simulink model "E3"  (R2020a)
settings: Solver=VariableStepAuto  StartTime=0.0  StopTime=200  RelTol=1e-3
undefined symbols (not defined in the file): c_s, kd, ki, kp
libraries: fl_lib x11, simulink x5, nesl_utility x5
settings Model: Creator=juan  LastModifiedBy=juan

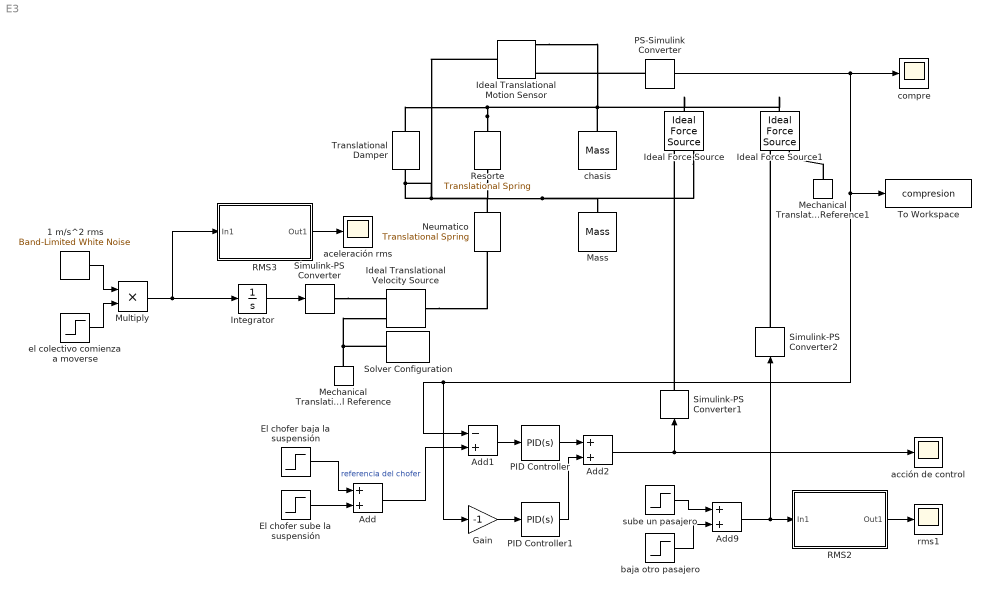
== system E3 ==
  1 m/s^2 rms : simulink/Sources/Band-Limited White Noise  Cov=(1^2)/(1/0.1)  Ts=0.1  seed=[98657]
  Add : Sum
  Add1 : Sum  Inputs=-+
  Add2 : Sum
  Add9 : Sum
  El chofer baja la suspensión : Step  Time=10  After=-0.10  SampleTime=0
  El chofer sube la suspensión : Step  Time=30  After=.10  SampleTime=0
  Gain : Gain  Gain=-1
  Ideal Force Source : fl_lib/Mechanical/Mechanical Sources/Ideal Force Source
  Ideal Force Source1 : fl_lib/Mechanical/Mechanical Sources/Ideal Force Source
  Ideal Translational Motion Sensor : fl_lib/Mechanical/Mechanical Sensors/Ideal Translational Motion Sensor  offset=0 m
  Ideal Translational Velocity Source : fl_lib/Mechanical/Mechanical Sources/Ideal Translational Velocity Source
  Integrator : Integrator
  Mass : fl_lib/Mechanical/Translational Elements/Mass  mass=m_u kg  v_specify=off  v_priority=High  v=0 m/s  v_nominal_specify=off  v_nominal_unit=m/s  v_nominal_value=1  f_specify=off  f_priority=None  f=0 N  f_nominal_specify=off  f_nominal_unit=N  f_nominal_value=1
  Mechanical Translational Reference : fl_lib/Mechanical/Translational Elements/Mechanical Translational Reference
  Mechanical Translational Reference1 : fl_lib/Mechanical/Translational Elements/Mechanical Translational Reference
  Multiply : Product
  Neumatico : fl_lib/Mechanical/Translational Elements/Translational Spring  spr_rate=k_t N/m  v_specify=off  v_priority=None  v=0 m/s  v_nominal_specify=off  v_nominal_unit=m/s  v_nominal_value=1  f_specify=off  f_priority=None  f=0 N  f_nominal_specify=off  f_nominal_unit=N  f_nominal_value=1  x_specify=off  x_priority=High  x=0 m  x_nominal_specify=off  x_nominal_unit=m  x_nominal_value=1
  PID Controller : simulink/Continuous/PID Controller  Controller=PID  Form=Parallel  TimeDomain=Continuous-time  UseExternalTs=off  SampleTime=-1  IntegratorMethod=Forward Euler  FilterMethod=Forward Euler  ControllerParametersSource=internal  P=0  I=ki  D=0  UseFilter=on  N=100  TunerSelectOption=Transfer Function Based (PID Tuner App)  InitialConditionSource=internal  InitialConditionForIntegrator=0  InitialConditionForFilter=0  DifferentiatorICPrevScaledInput=0  ExternalReset=none  TrackingMode=off  Kt=1  LimitOutput=off  UpperSaturationLimit=inf  LowerSaturationLimit=-inf  LinearizeAsGain=on  AntiWindupMode=none  Kb=1  POutMin=[]  POutMax=[]  IOutMin=[]  IOutMax=[]  DOutMin=[]  DOutMax=[]  NOutMin=[]  NOutMax=[]  SumOutMin=[]  SumOutMax=[]  SaturationOutMin=[]  SaturationOutMax=[]  PParamMin=[]  PParamMax=[]  IParamMin=[]  IParamMax=[]  DParamMin=[]  DParamMax=[]  NParamMin=[]  NParamMax=[]  KbParamMin=[]  KbParamMax=[]  KtParamMin=[]  KtParamMax=[]  KbOutMin=[]  KbOutMax=[]  KtOutMin=[]  KtOutMax=[]  IntegratorOutMin=[]  IntegratorOutMax=[]  FilterOutMin=[]  FilterOutMax=[]  SumI1OutMin=[]  SumI1OutMax=[]  SumI2OutMin=[]  SumI2OutMax=[]  SumI3OutMin=[]  SumI3OutMax=[]  SumI4OutMin=[]  SumI4OutMax=[]  SumDOutMin=[]  SumDOutMax=[]  DifferentiatorOutMin=[]  DifferentiatorOutMax=[]  FilterDiffOutCoefMin=[]  FilterDiffOutCoefMax=[]  ReciprocalOutMin=[]  ReciprocalOutMax=[]  SumDenOutMin=[]  SumDenOutMax=[]  SumNumOutMin=[]  SumNumOutMax=[]  DivideOutMin=[]  DivideOutMax=[]  UdiffTsProdOutMin=[]  UdiffTsProdOutMax=[]  NTsProdOutMin=[]  NTsProdOutMax=[]  UintegralTsProdOutMin=[]  UintegralTsProdOutMax=[]  UngainTsProdOutMin=[]  UngainTsProdOutMax=[]  IntegratorContinuousStateAttributes=''  IntegratorStateMustResolveToSignalObject=off  IntegratorRTWStateStorageClass=Auto  FilterContinuousStateAttributes=''  FilterStateMustResolveToSignalObject=off  FilterRTWStateStorageClass=Auto  ParallelPVariant=InternalParameters  IdealPVariant=Disabled  IVariant=InternalParameters  DVariant=InternalParameters  IntegratorVariant=Continuous  SatVariant=Disabled  AWVariant=Passthrough  PCopyVariant=Disabled  TRVariant=Disabled  FdbkBlocksVariant=Forward  IdealPFdbkVariant=Disabled  SatFdbkVariant=Disabled  DerivativeFilterVariant=ContFilter  NVariant=InternalParameters  NCopyVariant=Disabled  FilterICVariant=InternalICsFilter  IntegratorICVariant=InternalICs  ExternalResetVariant=Disabled  TRSumVariant=Passthrough  SumFdbkVariant=Disabled  SumVariant=Sum_PID  TsampFilterVariant=InternalTs  TsampNgainVariant=Passthrough  TsampIntegralVariant=Passthrough
  PID Controller1 : simulink/Continuous/PID Controller  Controller=PID  Form=Parallel  TimeDomain=Continuous-time  UseExternalTs=off  SampleTime=-1  IntegratorMethod=Forward Euler  FilterMethod=Forward Euler  ControllerParametersSource=internal  P=kp  I=0  D=kd  UseFilter=on  N=100  TunerSelectOption=Transfer Function Based (PID Tuner App)  InitialConditionSource=internal  InitialConditionForIntegrator=0  InitialConditionForFilter=0  DifferentiatorICPrevScaledInput=0  ExternalReset=none  TrackingMode=off  Kt=1  LimitOutput=off  UpperSaturationLimit=inf  LowerSaturationLimit=-inf  LinearizeAsGain=on  AntiWindupMode=none  Kb=1  POutMin=[]  POutMax=[]  IOutMin=[]  IOutMax=[]  DOutMin=[]  DOutMax=[]  NOutMin=[]  NOutMax=[]  SumOutMin=[]  SumOutMax=[]  SaturationOutMin=[]  SaturationOutMax=[]  PParamMin=[]  PParamMax=[]  IParamMin=[]  IParamMax=[]  DParamMin=[]  DParamMax=[]  NParamMin=[]  NParamMax=[]  KbParamMin=[]  KbParamMax=[]  KtParamMin=[]  KtParamMax=[]  KbOutMin=[]  KbOutMax=[]  KtOutMin=[]  KtOutMax=[]  IntegratorOutMin=[]  IntegratorOutMax=[]  FilterOutMin=[]  FilterOutMax=[]  SumI1OutMin=[]  SumI1OutMax=[]  SumI2OutMin=[]  SumI2OutMax=[]  SumI3OutMin=[]  SumI3OutMax=[]  SumI4OutMin=[]  SumI4OutMax=[]  SumDOutMin=[]  SumDOutMax=[]  DifferentiatorOutMin=[]  DifferentiatorOutMax=[]  FilterDiffOutCoefMin=[]  FilterDiffOutCoefMax=[]  ReciprocalOutMin=[]  ReciprocalOutMax=[]  SumDenOutMin=[]  SumDenOutMax=[]  SumNumOutMin=[]  SumNumOutMax=[]  DivideOutMin=[]  DivideOutMax=[]  UdiffTsProdOutMin=[]  UdiffTsProdOutMax=[]  NTsProdOutMin=[]  NTsProdOutMax=[]  UintegralTsProdOutMin=[]  UintegralTsProdOutMax=[]  UngainTsProdOutMin=[]  UngainTsProdOutMax=[]  IntegratorContinuousStateAttributes=''  IntegratorStateMustResolveToSignalObject=off  IntegratorRTWStateStorageClass=Auto  FilterContinuousStateAttributes=''  FilterStateMustResolveToSignalObject=off  FilterRTWStateStorageClass=Auto  ParallelPVariant=InternalParameters  IdealPVariant=Disabled  IVariant=InternalParameters  DVariant=InternalParameters  IntegratorVariant=Continuous  SatVariant=Disabled  AWVariant=Passthrough  PCopyVariant=Disabled  TRVariant=Disabled  FdbkBlocksVariant=Forward  IdealPFdbkVariant=Disabled  SatFdbkVariant=Disabled  DerivativeFilterVariant=ContFilter  NVariant=InternalParameters  NCopyVariant=Disabled  FilterICVariant=InternalICsFilter  IntegratorICVariant=InternalICs  ExternalResetVariant=Disabled  TRSumVariant=Passthrough  SumFdbkVariant=Disabled  SumVariant=Sum_PID  TsampFilterVariant=InternalTs  TsampNgainVariant=Passthrough  TsampIntegralVariant=Passthrough
  PS-Simulink Converter : nesl_utility/PS-Simulink Converter  PhysicalDomain=network_engine_domain  SubClassName=ps_output  LeftPortType=input  RightPortType=output  PseudoPeriodic=off  Frequencies=[]  Unit=1  AffineConversion=off
  RMS2 : Subsystem
  RMS3 : Subsystem
  Resorte : fl_lib/Mechanical/Translational Elements/Translational Spring  spr_rate=k_s N/m  v_specify=off  v_priority=None  v=0 m/s  v_nominal_specify=off  v_nominal_unit=m/s  v_nominal_value=1  f_specify=off  f_priority=None  f=0 N  f_nominal_specify=off  f_nominal_unit=N  f_nominal_value=1  x_specify=off  x_priority=High  x=0 m  x_nominal_specify=off  x_nominal_unit=m  x_nominal_value=1
  Simulink-PS Converter : nesl_utility/Simulink-PS Converter  PhysicalDomain=network_engine_domain  SubClassName=ps_input  LeftPortType=input  RightPortType=output  PseudoPeriodic=off  Frequencies=[]  NoiseDistribution=none  NoiseParameters=[]  Unit=1  AffineConversion=off  FilteringAndDerivatives=provide  SimscapeFilterOrder=1  InputFilterTimeConstant=0.001  UdotUserProvided=0
  Simulink-PS Converter1 : nesl_utility/Simulink-PS Converter  PhysicalDomain=network_engine_domain  SubClassName=ps_input  LeftPortType=input  RightPortType=output  PseudoPeriodic=off  Frequencies=[]  NoiseDistribution=none  NoiseParameters=[]  Unit=1  AffineConversion=off  FilteringAndDerivatives=provide  SimscapeFilterOrder=1  InputFilterTimeConstant=0.001  UdotUserProvided=0
  Simulink-PS Converter2 : nesl_utility/Simulink-PS Converter  PhysicalDomain=network_engine_domain  SubClassName=ps_input  LeftPortType=input  RightPortType=output  PseudoPeriodic=off  Frequencies=[]  NoiseDistribution=none  NoiseParameters=[]  Unit=1  AffineConversion=off  FilteringAndDerivatives=provide  SimscapeFilterOrder=1  InputFilterTimeConstant=0.001  UdotUserProvided=0
  Solver Configuration : nesl_utility/Solver Configuration  PhysicalDomain=network_engine_domain  SubClassName=solver  LeftPortType=input  RightPortType=generic  Tones=[]  Harmonics=[]  SimulateNoise=off  Profile=off  UseLocalSampling=off  EnableSwitchedLinearOptims=on  FrequencyDomain=off  UseCCode=off  RelTol=0.001  AbsTol=1e-06  MinStep=1e-09  ToWorkspace=off  RevertToSquareIcSolve=off  NumHomotopyIterations=100  PhasorMode=off  PhasorModeNumHarmonics=1  DoDC=off  ResidualTolerance=1e-09  UseLocalSolver=off  LocalSolverChoice=NE_BACKWARD_EULER_ADVANCER  LocalSolverSampleTime=0.001  DoFixedCost=off  MaxNonlinIter=3  MaxModeIter=2  LinearAlgebra=Sparse  EquationFormulation=NE_TIME_EF  DelaysMemoryBudget=1024  AutomaticFiltering=on  FilteringTimeConstant=0.001  PartitionStorageMethod=AS_NEEDED  PartitionMemoryBudget=1024  PartitionMethod=FAST
  To Workspace : ToWorkspace  VariableName=compresion  SaveFormat=Structure With Time  SampleTime=-1
  Translational Damper : fl_lib/Mechanical/Translational Elements/Translational Damper  D=c_s N/(m/s)  v_specify=off  v_priority=None  v=0 m/s  v_nominal_specify=off  v_nominal_unit=m/s  v_nominal_value=1  f_specify=off  f_priority=None  f=0 N  f_nominal_specify=off  f_nominal_unit=N  f_nominal_value=1
  acción de control : Scope
  aceleración rms : Scope
  baja otro pasajero : Step  Time=25  After=-700  SampleTime=0
  chasis : fl_lib/Mechanical/Translational Elements/Mass  mass=m_s kg  v_specify=off  v_priority=High  v=0 m/s  v_nominal_specify=off  v_nominal_unit=m/s  v_nominal_value=1  f_specify=off  f_priority=None  f=0 N  f_nominal_specify=off  f_nominal_unit=N  f_nominal_value=1
  compre : Scope
  el colectivo comienza a moverse : Step  Time=50  SampleTime=0
  rms1 : Scope
  sube un pasajero : Step  Time=20  After=700  SampleTime=0
  wires:
  El chofer sube la suspensión/1 -> Add/2
  Add/1 -> Add1/2  "referencia del chofer"
  sube un pasajero/1 -> Add9/1
  PS-Simulink Converter/1 -> To Workspace/1, Gain/1, Add1/1, compre/1
  Add1/1 -> PID Controller/1
  RMS2/1(Out1) -> rms1/1
  baja otro pasajero/1 -> Add9/2
  El chofer baja la suspensión/1 -> Add/1
  Add2/1 -> Simulink-PS Converter1/1, acción de control/1
  PID Controller/1 -> Add2/1
  Integrator/1 -> Simulink-PS Converter/1
  Multiply/1 -> Integrator/1, RMS3/1(In1)
  1 m/s^2 rms/1 -> Multiply/1
  Add9/1 -> RMS2/1(In1), Simulink-PS Converter2/1
  el colectivo comienza a moverse/1 -> Multiply/2
  RMS3/1(Out1) -> aceleración rms/1
  PID Controller1/1 -> Add2/2
  Gain/1 -> PID Controller1/1
  connections:
  Resorte/LConn1 -- chasis/LConn1 -- Ideal Force Source1/LConn1 -- Ideal Force Source/LConn1 -- Ideal Translational Motion Sensor/RConn1 -- Translational Damper/LConn1
  Translational Damper/RConn1 -- Neumatico/LConn1 -- Ideal Force Source/RConn2 -- Mass/LConn1 -- Resorte/RConn1 -- Ideal Translational Motion Sensor/LConn1
  Solver Configuration/RConn1 -- Ideal Translational Velocity Source/RConn2 -- Mechanical Translational Reference/LConn1
  Mechanical Translational Reference1/LConn1 -- Ideal Force Source1/RConn2
  Ideal Translational Velocity Source/LConn1 -- Neumatico/RConn1
  Simulink-PS Converter1/RConn1 -- Ideal Force Source/RConn1
  Simulink-PS Converter2/RConn1 -- Ideal Force Source1/RConn1
  PS-Simulink Converter/LConn1 -- Ideal Translational Motion Sensor/RConn3
  Simulink-PS Converter/RConn1 -- Ideal Translational Velocity Source/RConn1

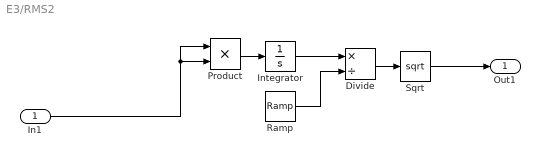
== system E3/RMS2 ==
  In1 : Inport
  Divide : Product  Inputs=*/
  Integrator : Integrator
  Product : Product
  Ramp : simulink/Sources/Ramp  slope=1  start=0  InitialOutput=0
  Sqrt : Sqrt  SaturateOnIntegerOverflow=on
  Out1 : Outport  VectorParamsAs1DForOutWhenUnconnected=off
  wires:
  Ramp/1 -> Divide/2
  Product/1 -> Integrator/1
  Integrator/1 -> Divide/1
  Sqrt/1 -> Out1/1
  Divide/1 -> Sqrt/1
  In1/1 -> Product/1, Product/2

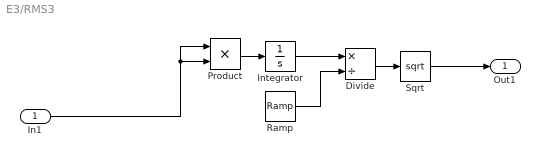
== system E3/RMS3 ==
  In1 : Inport
  Divide : Product  Inputs=*/
  Integrator : Integrator
  Product : Product
  Ramp : simulink/Sources/Ramp  slope=1  start=0  InitialOutput=0
  Sqrt : Sqrt  SaturateOnIntegerOverflow=on
  Out1 : Outport  VectorParamsAs1DForOutWhenUnconnected=off
  wires:
  Ramp/1 -> Divide/2
  Product/1 -> Integrator/1
  Integrator/1 -> Divide/1
  Sqrt/1 -> Out1/1
  Divide/1 -> Sqrt/1
  In1/1 -> Product/1, Product/2
